simulink model "RArsinus"  (Simulink 7.8)
settings: Solver=FixedStepDiscrete  StartTime=0.0  StopTime=30  FixedStep=1/(1024*4)  RelTol=1e-3
settings Model: Creator=root  LastModifiedBy=root  SimulationMode=external
settings DataIOCC: Decimation=5  LimitDataPoints=off
settings OptimizationCC: InitFltsAndDblsToZero=on
settings DebuggingCC: SolverPrmCheckMsg=none  FcnCallInpInsideContextMsg=Use local settings  UnconnectedInputMsg=none  UnconnectedOutputMsg=none  UnconnectedLineMsg=none  StrictBusMsg=Warning
settings RTWCC: SystemTargetFile=ectarget.tlc  MakeCommand="make_rtw OPTS=\"-DNETIF_ID=2\""  TemplateMakefile=ec_unix.tmf  Description=EtherCAT Real-Time Target for SOEM  RTWVerbose=off  ProcessScript=ectarget_make_rtw_hook
settings GRTTargetCC: ExtMode=on

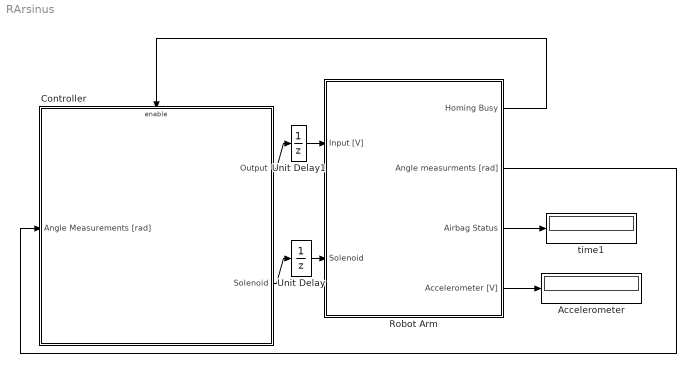
== system RArsinus ==
  Accelerometer : Display
      settings: Decimation=50
  Controller : Subsystem
  Robot Arm : Subsystem
      mask Description:
      | Hardware: Brom Mechatronica
      | Software: Victor Dolk
      mask Help: eval('feval(''rtwprivate'',''rtwhelpview'',''rtw_sfcn_block'')');
      mask Display:
      | image(imread('RobotArm.png'))
      | color('red');port_label('output', 1, 'Homing Busy')
      | port_label('output', 2, 'Angle Measurements')
      | port_label('output', 3, 'Airbag Status')
      | port_label('output', 4, 'Accelerometer [V]')
      | port_label('input', 1, 'Input [V]')
      | port_label('input', 2, 'Solenoid')
  Unit Delay : UnitDelay  SampleTime=-1
  Unit Delay1 : UnitDelay  SampleTime=-1
  time1 : Display
      settings: Decimation=50
  wires:
  Controller/1(Output) -> Unit Delay1/1
  Robot Arm/1(Homing Busy) -> Controller/Enable
  Robot Arm/2(Angle measurments [rad]) -> Controller/1(Angle Measurements [rad])
  Robot Arm/3(Airbag Status) -> time1/1
  Robot Arm/4(Accelerometer [V]) -> Accelerometer/1
  Controller/2(Solenoid) -> Unit Delay/1
  Unit Delay/1 -> Robot Arm/2(Solenoid)
  Unit Delay1/1 -> Robot Arm/1(Input [V])

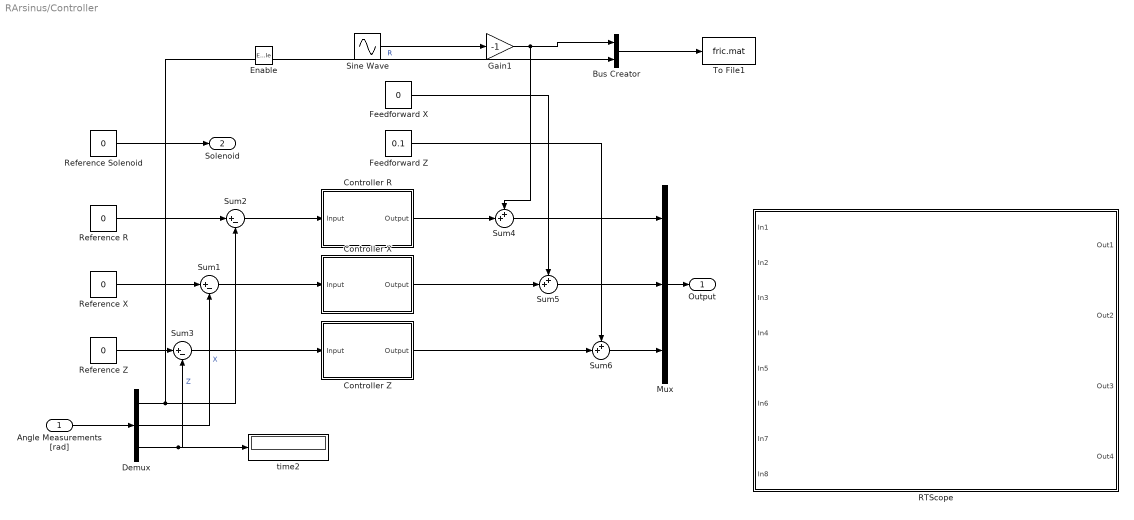
== system RArsinus/Controller ==
  Angle Measurements [rad] : Inport
  Enable : EnablePort
  Bus Creator : BusCreator  Inputs=2
  Controller R : Subsystem
  Controller X : Subsystem
  Controller Z : Subsystem
  Demux : Demux  Outputs=3
  Feedforward X : Constant  Value=0
  Feedforward Z : Constant  Value=0.1
  Gain1 : Gain  Gain=-1
  Mux : Mux  Inputs=3
  RTScope : Subsystem
      settings: OpenFcn=rtscope
      mask Type: RTScope
      mask Display: image(imread('rtscope2.jpg'))
  Reference R : Constant  Value=0
  Reference Solenoid : Constant  Value=0
  Reference X : Constant  Value=0
  Reference Z : Constant  Value=0
  Sine Wave : Sin  Amplitude=0.25  Frequency=12  SampleTime=0
  Sum1 : Sum  Inputs=|+-
  Sum2 : Sum  Inputs=|+-
  Sum3 : Sum  Inputs=|+-
  Sum4 : Sum  Inputs=++|  SaturateOnIntegerOverflow=on  InputSameDT=on  OutDataTypeStr=Inherit: Same as first input
  Sum5 : Sum  Inputs=++|  SaturateOnIntegerOverflow=on  InputSameDT=on  OutDataTypeStr=Inherit: Same as first input
  Sum6 : Sum  Inputs=++|  SaturateOnIntegerOverflow=on  InputSameDT=on  OutDataTypeStr=Inherit: Same as first input
  To File1 : ToFile  Filename=fric.mat  MatrixName=fric_stat
  time2 : Display
      settings: Decimation=50
  Output : Outport
  Solenoid : Outport  Port=2  InitialOutput=0
  wires:
  Mux/1 -> Output/1
  Angle Measurements [rad]/1 -> Demux/1
  Sum2/1 -> Controller R/1(Input)
  Sum3/1 -> Controller Z/1(Input)
  Sum1/1 -> Controller X/1(Input)
  Demux/1 -> Sum2/2, Bus Creator/2  "R"
  Demux/2 -> Sum1/2  "X"
  Demux/3 -> Sum3/2, time2/1  "Z"
  Controller R/1(Output) -> Sum4/2
  Sum4/1 -> Mux/1
  Feedforward X/1 -> Sum5/1
  Controller X/1(Output) -> Sum5/2
  Sum5/1 -> Mux/2
  Controller Z/1(Output) -> Sum6/2
  Sum6/1 -> Mux/3
  Feedforward Z/1 -> Sum6/1
  Reference R/1 -> Sum2/1
  Reference X/1 -> Sum1/1
  Reference Z/1 -> Sum3/1
  Reference Solenoid/1 -> Solenoid/1
  Bus Creator/1 -> To File1/1
  Gain1/1 -> Bus Creator/1, Sum4/1
  Sine Wave/1 -> Gain1/1

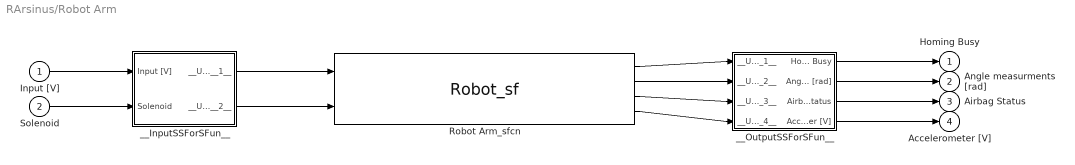
== system RArsinus/Robot Arm ==
  Input [V] : Inport
  Solenoid : Inport  Port=2
  Robot Arm_sfcn : S-Function  FunctionName=Robot_sf  SFunctionModules=ec_Ebox dweakint dpd dnotch dlowpass2 ec_EboxResetEnc  EnableBusSupport=off  mask{rtw_sf_name=Robot_sf, showVar=off}
      mask prompts: rtw_sf_name "Generated S-function name (model_sf):"; showVar "Show module list"
      mask help: Simulink Coder generated S-function.
      mask init:
      | displist = '';
      | if ~strcmp(get_param(gcb, 'FunctionName'), rtw_sf_name);
      |   set_param(gcb, 'FunctionName', rtw_sf_name);
      | end
      | % Check if we are generating code
      | rtw_mode = false;
      | if strcmpi(get_param(bdroot(gcb),'SimulationStatus'),'Initializing')
      | 	rtw_mode = strcmpi(get_param(bdroot(gcb),'BuildingRTWCode'),'on') && ...
      | 		~strcmpi(get_param(bdroot(gcb),'TargetStyle'),'SimulationTarget');
      | end
      | if showVar || rtw_mode
      | 	if exist('rtwsfunc') == 2 | exist('rtwsfunc') == 6
      | 		tmplist = rtwsfunc(rtw_sf_name,gcb);
      | 		tmplist = ['\nList of Modules:\n', tmplist];
      | 	elseif showVar
      | 		tmplist = '\nList of Modules:\nNot licensed\n';
      |  	end
      | end
      | if showVar
      |   displist = tmplist;
      | end
      settings: CopyFcn=|
      | if ~strcmp(get_param(gcb,'Linkstatus'),'none') && ...
      | ~strcmp(get_param(gcb,'Linkstatus'),'implicit')
      |   set_param(gcb,'LinkStatus','none');
      | end
      mask Help: eval('feval(''rtwprivate'',''rtwhelpview'',''rtw_sfcn_block'')');
      mask Display:
      | port_label('input',1,'Input [V]');
      | port_label('input',2,'Solenoid');
      | port_label('output',1,'Homing Busy');
      | port_label('output',2,'Angle measurments [rad]');
      | port_label('output',3,'Airbag Status');
      | port_label('output',4,'Accelerometer [V]');
  __InputSSForSFun__ : Subsystem
  __OutputSSForSFun__ : Subsystem
  Homing Busy : Outport
  Angle measurments [rad] : Outport  Port=2
  Airbag Status : Outport  Port=3
  Accelerometer [V] : Outport  Port=4
  wires:
  Input [V]/1 -> __InputSSForSFun__/1(Input [V])
  Solenoid/1 -> __InputSSForSFun__/2(Solenoid)
  __InputSSForSFun__/1(__UniqueOutportName__1__) -> Robot Arm_sfcn/1
  __InputSSForSFun__/2(__UniqueOutportName__2__) -> Robot Arm_sfcn/2
  Robot Arm_sfcn/1 -> __OutputSSForSFun__/1(__UniqueInportName__1__)
  Robot Arm_sfcn/2 -> __OutputSSForSFun__/2(__UniqueInportName__2__)
  Robot Arm_sfcn/3 -> __OutputSSForSFun__/3(__UniqueInportName__3__)
  Robot Arm_sfcn/4 -> __OutputSSForSFun__/4(__UniqueInportName__4__)
  __OutputSSForSFun__/1(Homing Busy) -> Homing Busy/1
  __OutputSSForSFun__/2(Angle measurments [rad]) -> Angle measurments [rad]/1
  __OutputSSForSFun__/3(Airbag Status) -> Airbag Status/1
  __OutputSSForSFun__/4(Accelerometer [V]) -> Accelerometer [V]/1

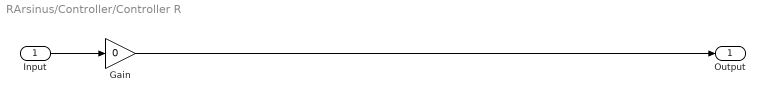
== system RArsinus/Controller/Controller R ==
  Input : Inport
  Gain : Gain  Gain=0
  Output : Outport
  wires:
  Input/1 -> Gain/1
  Gain/1 -> Output/1

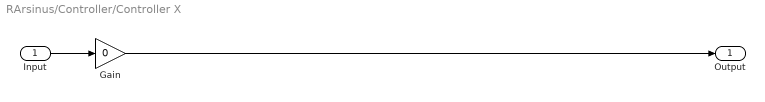
== system RArsinus/Controller/Controller X ==
  Input : Inport
  Gain : Gain  Gain=0
  Output : Outport
  wires:
  Gain/1 -> Output/1
  Input/1 -> Gain/1

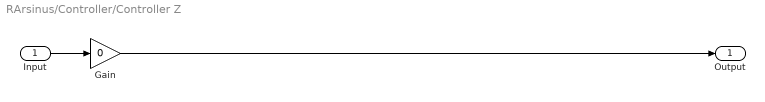
== system RArsinus/Controller/Controller Z ==
  Input : Inport
  Gain : Gain  Gain=0
  Output : Outport
  wires:
  Input/1 -> Gain/1
  Gain/1 -> Output/1

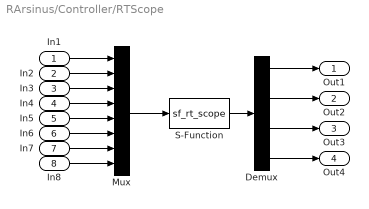
== system RArsinus/Controller/RTScope ==
  In1 : Inport
  In2 : Inport  Port=2
  In3 : Inport  Port=3
  In4 : Inport  Port=4
  In5 : Inport  Port=5
  In6 : Inport  Port=6
  In7 : Inport  Port=7
  In8 : Inport  Port=8
  Demux : Demux
  Mux : Mux  Inputs=8
  S-Function : S-Function  FunctionName=sf_rt_scope  Parameters=4096  EnableBusSupport=off
  Out1 : Outport
  Out2 : Outport  Port=2
  Out3 : Outport  Port=3
  Out4 : Outport  Port=4
  wires:
  In8/1 -> Mux/8
  In7/1 -> Mux/7
  In6/1 -> Mux/6
  In5/1 -> Mux/5
  In4/1 -> Mux/4
  In3/1 -> Mux/3
  In2/1 -> Mux/2
  In1/1 -> Mux/1
  Demux/4 -> Out4/1
  Demux/3 -> Out3/1
  Demux/2 -> Out2/1
  Demux/1 -> Out1/1
  S-Function/1 -> Demux/1
  Mux/1 -> S-Function/1

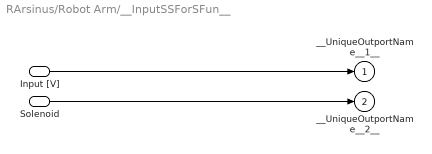
== system RArsinus/Robot Arm/__InputSSForSFun__ ==
  Input [V] : Inport
  Solenoid : Inport  Port=2
  __UniqueOutportName__1__ : Outport
  __UniqueOutportName__2__ : Outport  Port=2
  wires:
  Input [V]/1 -> __UniqueOutportName__1__/1
  Solenoid/1 -> __UniqueOutportName__2__/1

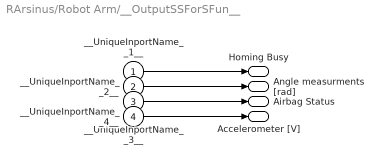
== system RArsinus/Robot Arm/__OutputSSForSFun__ ==
  __UniqueInportName__1__ : Inport
  __UniqueInportName__2__ : Inport  Port=2
  __UniqueInportName__3__ : Inport  Port=3
  __UniqueInportName__4__ : Inport  Port=4
  Homing Busy : Outport
  Angle measurments [rad] : Outport  Port=2
  Airbag Status : Outport  Port=3
  Accelerometer [V] : Outport  Port=4
  wires:
  __UniqueInportName__1__/1 -> Homing Busy/1
  __UniqueInportName__2__/1 -> Angle measurments [rad]/1
  __UniqueInportName__3__/1 -> Airbag Status/1
  __UniqueInportName__4__/1 -> Accelerometer [V]/1
